simulink model "simu_21uec072"  (R2022b)
settings: Solver=VariableStepAuto  StartTime=0.0  StopTime=0  RelTol=1e-3
settings Model: Creator=DSP-27  LastModifiedBy=DSP-27

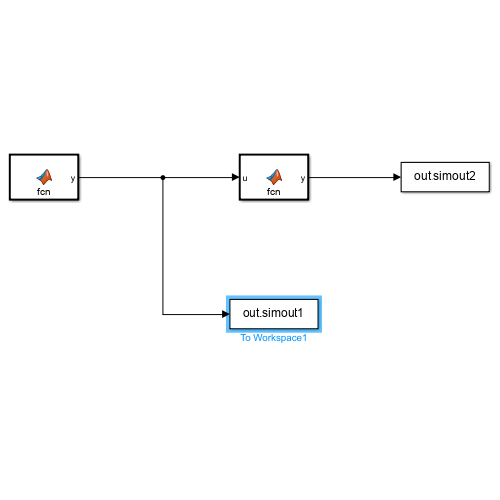
[thumbnail: Simulink's stored preview of the top-level diagram]
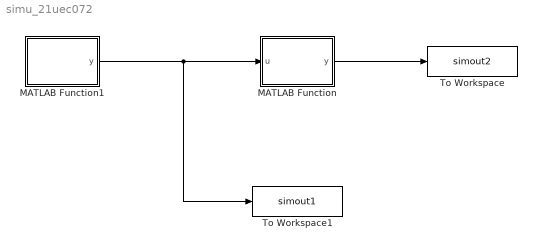
== system simu_21uec072 ==
  MATLAB Function : MATLAB Function  TreatAsAtomicUnit=on
  MATLAB Function1 : MATLAB Function  TreatAsAtomicUnit=on
  To Workspace : ToWorkspace  VariableName=simout2  SampleTime=-1
      settings: Save2DSignal=2-D array (concatenate along first dimension)
  To Workspace1 : ToWorkspace  VariableName=simout1  SampleTime=-1
      settings: Save2DSignal=2-D array (concatenate along first dimension)
  wires:
  MATLAB Function1/1(y) -> To Workspace1/1, MATLAB Function/1(u)
  MATLAB Function/1(y) -> To Workspace/1

== matlab function simu_21uec072/MATLAB Function ==
  data: u input; y output
function y = fcn(u)

coder.extrinsic('dct')
coder.extrinsic('idct')

y = zeros(1, length(u));
z = zeros(1, length(u));
y = dct(u);
z = idct(y);

y = z;

== matlab function simu_21uec072/MATLAB Function1 ==
  data: y output
function y = fcn()

y = zeros(1, 10000);
coder.extrinsic('audioread');
[audio,~] = audioread('handel.wav', [1, 10000]);

y = audio';
end
